simulink model "ntnu_leg_pos_mpc"  (R2022b)
settings: Solver=VariableStepAuto  StartTime=0.0  StopTime=3  MaxStep=1e-3  RelTol=1e-3  AbsTol=1e-6
undefined symbols (not defined in the file): lbu_sim, nx, ubu_sim, xref_tc, y_ref, y_ref_sim
settings Model: Creator=papaveneti  LastModifiedBy=papaveneti

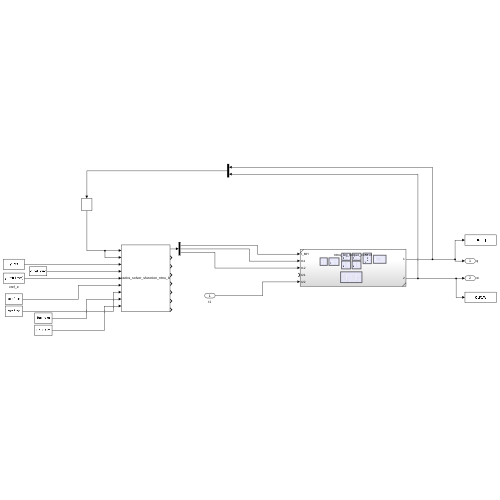
[thumbnail: Simulink's stored preview of the top-level diagram]
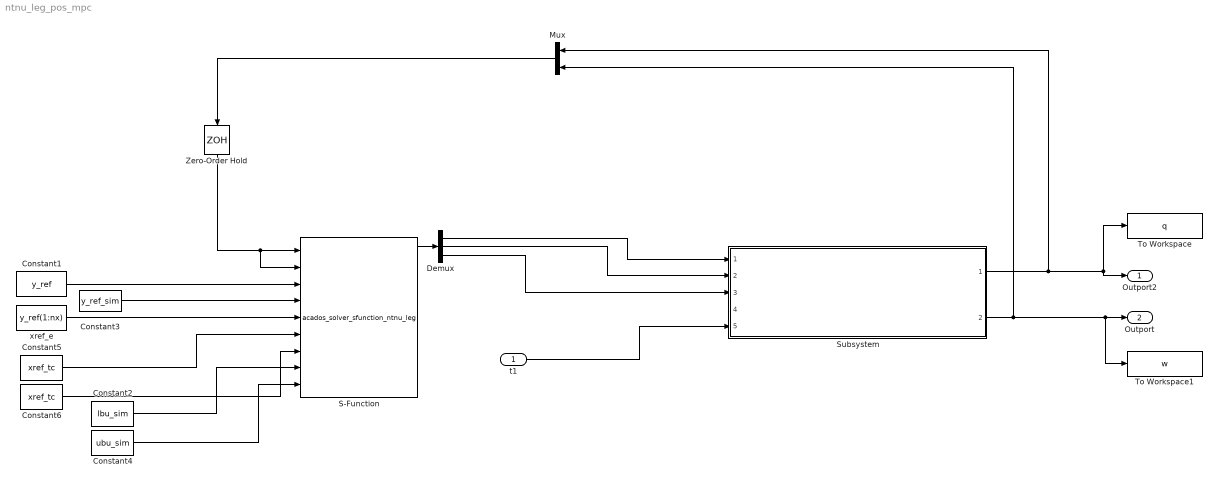
== system ntnu_leg_pos_mpc ==
  t1 : Inport
  Constant1 : Constant  Value=y_ref
  Constant2 : Constant  Value=lbu_sim
  Constant3 : Constant  Value=y_ref_sim
  Constant4 : Constant  Value=ubu_sim
  Constant5 : Constant  Value=xref_tc
  Constant6 : Constant  Value=xref_tc
  Demux : Demux  Outputs=3
  Mux : Mux  Inputs=2
  S-Function : S-Function  FunctionName=acados_solver_sfunction_ntnu_leg  SFunctionDeploymentMode=off  EnableBusSupport=off
  Subsystem : Subsystem  ReferencedSubsystem=ntnu_leg_torque_control
  To Workspace : ToWorkspace  VariableName=q  SaveFormat=Timeseries  SampleTime=-1
  To Workspace1 : ToWorkspace  VariableName=w  SaveFormat=Timeseries  SampleTime=-1
  Zero-Order Hold : ZeroOrderHold  SampleTime=1e-2
  xref_e : Constant  Value=y_ref(1:nx)
  Outport2 : Outport  SignalName=q
  Outport : Outport  Port=2  SignalName=w
  wires:
  Demux/1 -> Subsystem/1
  Demux/2 -> Subsystem/2
  t1/1 -> Subsystem/5
  Subsystem/1 -> Mux/1, Outport2/1, To Workspace/1
  Subsystem/2 -> Mux/2, To Workspace1/1, Outport/1
  Constant3/1 -> S-Function/4
  xref_e/1 -> S-Function/5
  Constant1/1 -> S-Function/3
  Constant4/1 -> S-Function/9
  Constant2/1 -> S-Function/8
  Constant5/1 -> S-Function/6
  Constant6/1 -> S-Function/7
  S-Function/1 -> Demux/1
  Mux/1 -> Zero-Order Hold/1
  Zero-Order Hold/1 -> S-Function/2, S-Function/1
  Demux/3 -> Subsystem/3
